simulink model "part2"  (R2022b)
settings: Solver=FixedStepAuto  StartTime=0.0  StopTime=500  FixedStep=0.1  RelTol=1e-3
values from neighbouring files (symbols this model uses):
  beta_c = 270    [init.m]
  D = [2.6486e5 0 0; 0 8.8164e5 0; 0 0 3.3774e8]    [KalmanKladd.m]    (also in init.m)
  init_setPoint = [0 0 0]    [init.m]
  K1 = [diag([k_1,k_2,k_3]) ... (first row only)    [init.m]
  K2 = diag([k_7,k_8,k_9])    [init.m]
  K3 = 0.05*K4    [init.m]
  K4 = diag([diag(M)])    [init.m]
  Kd = [7e6 7e6 1e9]    [init.m]
  Ki = [1e3 3e5 1e6]    [init.m]
  Kp = [4e6 4e6 2e8]    [init.m]
  M = [6.8177e6 0 0; 0 7.8784e6 -2.5955e6; 0 -2.5955e6 3.57e9]    [KalmanKladd.m]    (also in init.m)
  omg2 = omg.*omg    [init.m]
  satMax = [3 3 0.05]    [init.m]
  setPoint0 = [0 0 0]    [init.m]
  setPoint1 = [50 0 0]    [init.m]
  setPoint2 = [50 -50 0]    [init.m]
  setPoint3 = [50 -50 -pi/4]    [init.m]
  setPoint4 = [0 -50 -pi/4]    [init.m]
  setPoint5 = [0 0 0]    [init.m]
  setPoint_change_time = 100    [init.m]
  setPoint_sim12 = [0 0 0]    [init.m]
  setPoint_sim3 = [10 10 3*pi/2]    [init.m]
  switch_condition = 0    [init.m]
  thrusters =     [thrusters_sup.mat]
  V_c = 0.2    [init.m]
  vessel =     [thrusters_sup.mat]
  Z2omg = 2*omg.*zeta    [init.m]
undefined symbols (not defined in the file or in its folder): A_w, C_w, Hoerner, T
libraries: marine_gnc x7, marine_hydro x2, simulink x1
settings Model: Creator=jonbjor  LastModifiedBy=Petter
settings SolverCC: AlgebraicLoopSolver=TrustRegion
settings DataIOCC: ReturnWorkspaceOutputs=off
settings DebuggingCC: UnconnectedInputMsg=warning  UnconnectedOutputMsg=warning  UnconnectedLineMsg=warning  SFMachineParentedDataDiag=warning  ArithmeticOperatorsInVariantConditions=warning
settings ModelReferenceCC: EnableRefExpFcnMdlSchedulingChecks=on
settings SFSimCC: SimUseLocalCustomCode=off  CustomCodeUndefinedFunction=UseInterfaceOnly
settings RTWCC: RTWUseLocalCustomCode=off

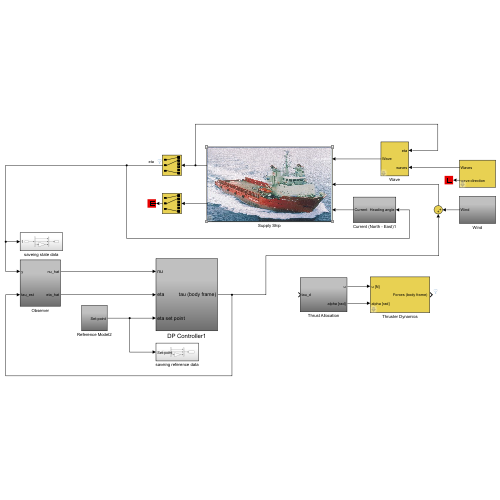
[thumbnail: Simulink's stored preview of the top-level diagram]
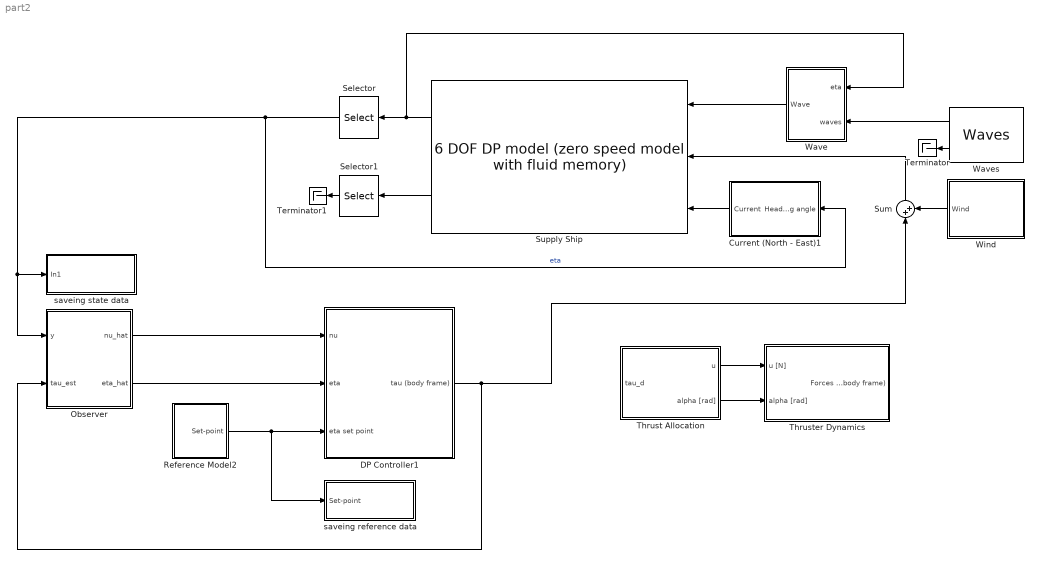
== system part2 ==
  Current (North - East)1 : Subsystem
  DP Controller1 : Subsystem
  Observer : Subsystem
  Reference Model2 : Subsystem
  Selector : Selector  InputPortWidth=6  IndexOptions=Index vector (dialog)  Indices=[1 2 6]  OutputSizes=1
  Selector1 : Selector  InputPortWidth=6  IndexOptions=Index vector (dialog)  Indices=[1 2 6]  OutputSizes=1
  Sum : Sum  Inputs=|++
  Supply Ship : marine_hydro/Hydro Library/6 DOF DP model  (zero speed model with fluid memory)  ABC=vesselABC  rho=1025  Axc=0.9*vessel.main.T*vessel.main.B  Ayc=0.9*vessel.main.T*vessel.main.Lpp  CX=1  CY_2D=Hoerner(vessel.main.B,vessel.main.T)  Bv=vessel.Bv  mask(6 DOF zero speed model){}
      link override "Integrator1 ": InitialCondition=nu0
      link override Integrator2: InitialCondition=eta0
      settings: SourceProductName=MSS Hydro
      mask Display:
      | image('supply.jpg');
      | color('white'); port_label('output', 1, 'eta')
      | color('white'); port_label('output', 2, 'nu')
      | color('white'); port_label('input', 1, 'tau_wave')
      | color('white'); port_label('input', 2, 'tau')
      | color('white'); port_label('input', 3, 'nu_c')
  Terminator : Terminator
  Terminator1 : Terminator
  Thrust Allocation : Subsystem
  Thruster Dynamics : Subsystem  mask{thrusterfault=off}
      mask prompts: thrusterfault "Fault on thruster #2 and #5?"
  Wave : Subsystem  mask{waveforces=on}
      mask prompts: waveforces "Waveforces enabled"
  Waves : marine_gnc/Environment/Waves/Waves  spectrum_type=ITTC  disp_flag=on  plot_spectrum=off  plot_realization=off  hs=5  omega_peak=pi/10  psi_mean=0  gamma=-1  spread=2  depth=inf  nfreq=20  ndir=10  energylim=0.005  freq_cutoff=3  dir_cutoff=0  rand_seed=123  rand_freq=on  rand_dir=on  Zeta_a=0  Omega=0  Phase=0  Wavenum=0  Psi=0
      settings: SourceProductName=MSS GNC
  Wind : Subsystem
  saveing reference data : Subsystem
  saveing state data : Subsystem
  wires:
  Supply Ship/2 -> Selector1/1
  Supply Ship/1 -> Wave/1(eta), Selector/1
  Wave/1(Wave) -> Supply Ship/1
  Waves/1 -> Wave/2(waves)
  Waves/2 -> Terminator/1
  Selector1/1 -> Terminator1/1
  Thrust Allocation/1(u) -> Thruster Dynamics/1(u [N])
  Wind/1(Wind) -> Sum/2
  DP Controller1/1(tau (body frame)) -> Observer/2(tau_est), Sum/1
  Sum/1 -> Supply Ship/2
  Thrust Allocation/2(alpha [rad]) -> Thruster Dynamics/2(alpha [rad])
  Selector/1 -> Current (North - East)1/1(Heading angle), saveing state data/1(In1), Observer/1(y)  "eta"
  Observer/2(eta_hat) -> DP Controller1/2(eta)
  Observer/1(nu_hat) -> DP Controller1/1(nu)
  Reference Model2/1(Set-point) -> saveing reference data/1(Set-point), DP Controller1/3(eta set point)
  Current (North - East)1/1(Current) -> Supply Ship/3

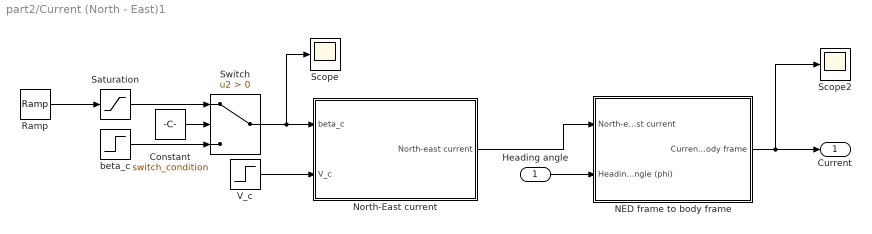
== system part2/Current (North - East)1 ==
  Heading angle : Inport
  Constant : Constant  Value=switch_condition
  NED frame to body frame : Subsystem
  North-East current : Subsystem
  Ramp : simulink/Sources/Ramp  slope=0.5  start=0  InitialOutput=0
  Saturation : Saturate  UpperLimit=90  LowerLimit=0
  Scope : Scope
  Scope2 : Scope
  Switch : Switch  Criteria=u2 > Threshold  SaturateOnIntegerOverflow=off  InputSameDT=off
  V_c : Step  Time=0  After=V_c  SampleTime=0
  beta_c : Step  Time=0  After=beta_c  SampleTime=0
  Current : Outport  VectorParamsAs1DForOutWhenUnconnected=off
  wires:
  V_c/1 -> North-East current/2(V_c)
  North-East current/1(North-east current) -> NED frame to body frame/1(North-east current)
  Heading angle/1 -> NED frame to body frame/2(Heading angle (phi))
  NED frame to body frame/1(Current body frame) -> Current/1, Scope2/1
  Ramp/1 -> Saturation/1
  Saturation/1 -> Switch/1
  Constant/1 -> Switch/2
  Switch/1 -> Scope/1, North-East current/1(beta_c)
  beta_c/1 -> Switch/3

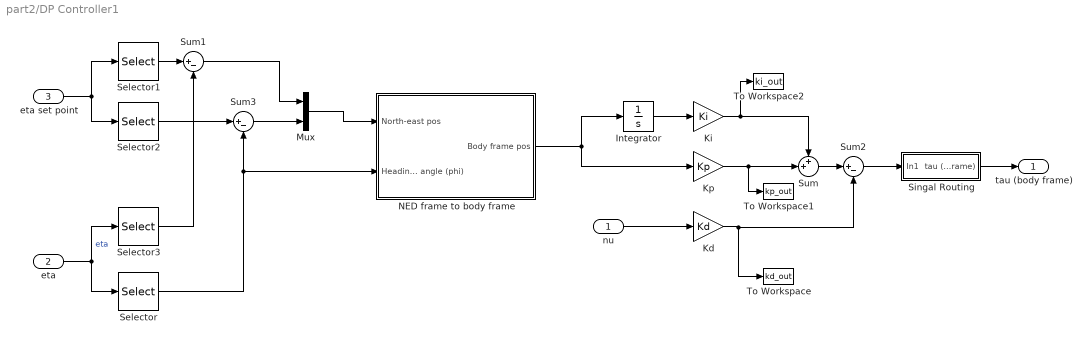
== system part2/DP Controller1 ==
  nu : Inport
  eta : Inport  Port=2
  eta set point : Inport  Port=3
  Integrator : Integrator
  Kd : Gain  Gain=Kd
  Ki : Gain  Gain=Ki
  Kp : Gain  Gain=Kp
  Mux : Mux  Inputs=2
  NED frame to body frame : Subsystem
  Selector : Selector  InputPortWidth=3  IndexOptions=Index vector (dialog)  Indices=[3]  OutputSizes=1
  Selector1 : Selector  InputPortWidth=3  IndexOptions=Index vector (dialog)  Indices=[1 2]  OutputSizes=1
  Selector2 : Selector  InputPortWidth=3  IndexOptions=Index vector (dialog)  Indices=[3]  OutputSizes=1
  Selector3 : Selector  InputPortWidth=3  IndexOptions=Index vector (dialog)  Indices=[1 2]  OutputSizes=1
  Singal Routing : Subsystem
  Sum : Sum  Inputs=++|
  Sum1 : Sum  Inputs=|+-
  Sum2 : Sum  Inputs=|+-
  Sum3 : Sum  Inputs=|+-
  To Workspace : ToWorkspace  VariableName=kd_out  SaveFormat=Timeseries  SampleTime=-1
  To Workspace1 : ToWorkspace  VariableName=kp_out  SaveFormat=Timeseries  SampleTime=-1
  To Workspace2 : ToWorkspace  VariableName=ki_out  SaveFormat=Timeseries  SampleTime=-1
  tau (body frame) : Outport  VectorParamsAs1DForOutWhenUnconnected=off
  wires:
  Kp/1 -> To Workspace1/1, Sum/2
  Ki/1 -> Sum/1, To Workspace2/1
  Kd/1 -> Sum2/2, To Workspace/1
  Integrator/1 -> Ki/1
  Sum/1 -> Sum2/1
  nu/1 -> Kd/1
  Sum2/1 -> Singal Routing/1(In1)
  Singal Routing/1(tau (body frame)) -> tau (body frame)/1
  NED frame to body frame/1(Body frame pos) -> Integrator/1, Kp/1
  eta set point/1 -> Selector2/1, Selector1/1
  eta/1 -> Selector/1, Selector3/1  "eta"
  Selector1/1 -> Sum1/1
  Selector3/1 -> Sum1/2
  Selector2/1 -> Sum3/1
  Selector/1 -> Sum3/2, NED frame to body frame/2(Heading angle (phi))
  Sum3/1 -> Mux/2
  Sum1/1 -> Mux/1
  Mux/1 -> NED frame to body frame/1(North-east pos)

== system part2/Observer ==
  y : Inport
  tau_est : Inport  Port=2
  Passive DP wave filter : marine_gnc/Navigation/Observers/Passive DP wave filter  lambda=0.1*diag([1 1 1])  w_o=diag([0.8 0.8 0.8])  K4=0.1*diag([1 1 0.1])  K3=0.1*diag([1 1 0.1])  w_c=1.3*diag([0.8 0.8 0.8])  T_b=diag([100 100 100])  M=diag([1 1 1])  D=diag([1 1 1])
      settings: SourceProductName=MSS GNC
  "Passive nonlinear observer " : Subsystem
  nu_hat : Outport  VectorParamsAs1DForOutWhenUnconnected=off
  eta_hat : Outport  Port=2  VectorParamsAs1DForOutWhenUnconnected=off
  wires:
  y/1 -> "Passive nonlinear observer "/1(y)
  tau_est/1 -> "Passive nonlinear observer "/2(tau_est)
  "Passive nonlinear observer "/1(nu_hat) -> nu_hat/1
  "Passive nonlinear observer "/2(eta_hat) -> eta_hat/1

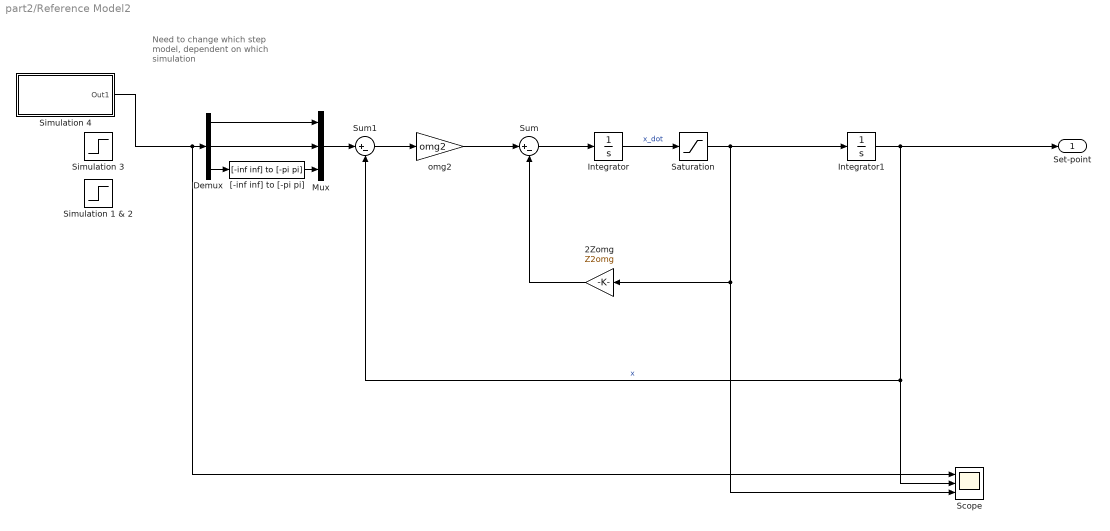
== system part2/Reference Model2 ==
  note: Need to change which step model, dependent on which simulation
  2Zomg : Gain  Gain=Z2omg
  Demux : Demux  Outputs=3
  Integrator : Integrator
  Integrator1 : Integrator
  Mux : Mux  Inputs=3
  Saturation : Saturate  UpperLimit=satMax  LowerLimit=-satMax
  Scope : Scope  NumInputPorts=3
  Simulation 1 & 2 : Step  Time=0  After=setPoint_sim12  SampleTime=0
  Simulation 3 : Step  Time=setPoint_change_time  Before=init_setPoint  After=setPoint_sim3  SampleTime=0
  Simulation 4 : Subsystem
  Sum : Sum  Inputs=|+-
  Sum1 : Sum  Inputs=|+-
  "[-inf inf] to [-pi pi]" : marine_gnc/Utilities/Math Operations/[-inf inf] to [-pi pi]
      settings: SourceProductName=MSS GNC
  omg2 : Gain  Gain=omg2
  Set-point : Outport  VectorParamsAs1DForOutWhenUnconnected=off
  wires:
  Integrator1/1 -> Set-point/1, Sum1/2, Scope/2  "x"
  Saturation/1 -> 2Zomg/1, Scope/3, Integrator1/1
  omg2/1 -> Sum/1
  Integrator/1 -> Saturation/1  "x_dot"
  Sum/1 -> Integrator/1
  Sum1/1 -> omg2/1
  2Zomg/1 -> Sum/2
  Simulation 4/1(Out1) -> Scope/1, Demux/1
  Mux/1 -> Sum1/1
  Demux/1 -> Mux/1
  Demux/2 -> Mux/2
  Demux/3 -> "[-inf inf] to [-pi pi]"/1
  "[-inf inf] to [-pi pi]"/1 -> Mux/3

== system part2/Thrust Allocation ==
  tau_d : Inport
  u : Outport  VectorParamsAs1DForOutWhenUnconnected=off
  alpha [rad] : Outport  Port=2  VectorParamsAs1DForOutWhenUnconnected=off

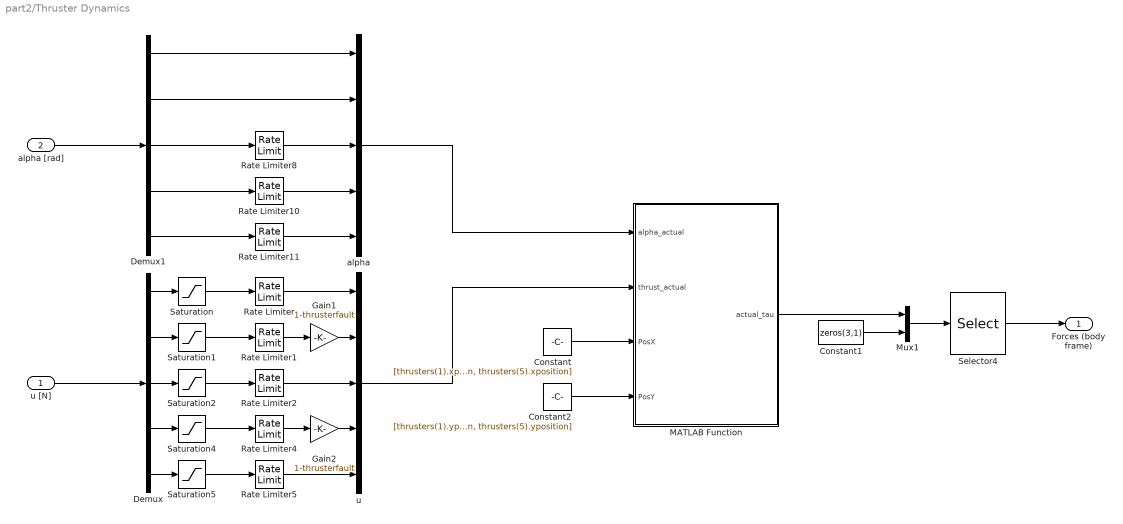
== system part2/Thruster Dynamics ==
  u [N] : Inport
  alpha [rad] : Inport  Port=2
  Constant : Constant  Value=[thrusters(1).xposition, thrusters(2).xposition, thrusters(3).xposition, thrusters(4).xposition, thrusters(5).xposition]
  Constant1 : Constant  Value=zeros(3,1)
  Constant2 : Constant  Value=[thrusters(1).yposition, thrusters(2).yposition, thrusters(3).yposition, thrusters(4).yposition, thrusters(5).yposition]
  Demux : Demux  Outputs=5
  Demux1 : Demux  Outputs=5
  Gain1 : Gain  Gain=1-thrusterfault
  Gain2 : Gain  Gain=1-thrusterfault
  MATLAB Function : MATLAB Function  TreatAsAtomicUnit=on
  Mux1 : Mux  Inputs=2
  Rate Limiter : RateLimiter  RisingSlewLimit=thrusters(1).rate  FallingSlewLimit=-thrusters(1).rate  SampleTimeMode=inherited
  Rate Limiter1 : RateLimiter  RisingSlewLimit=thrusters(2).rate  FallingSlewLimit=-thrusters(2).rate  SampleTimeMode=inherited
  Rate Limiter10 : RateLimiter  RisingSlewLimit=thrusters(4).rotationspeed  FallingSlewLimit=-thrusters(4).rotationspeed  SampleTimeMode=inherited
  Rate Limiter11 : RateLimiter  RisingSlewLimit=thrusters(5).rotationspeed  FallingSlewLimit=-thrusters(5).rotationspeed  SampleTimeMode=inherited
  Rate Limiter2 : RateLimiter  RisingSlewLimit=thrusters(3).rate  FallingSlewLimit=-thrusters(3).rate  SampleTimeMode=inherited
  Rate Limiter4 : RateLimiter  RisingSlewLimit=thrusters(4).rate  FallingSlewLimit=-thrusters(4).rate  SampleTimeMode=inherited
  Rate Limiter5 : RateLimiter  RisingSlewLimit=thrusters(5).rate  FallingSlewLimit=-thrusters(5).rate  SampleTimeMode=inherited
  Rate Limiter8 : RateLimiter  RisingSlewLimit=thrusters(3).rotationspeed  FallingSlewLimit=-thrusters(3).rotationspeed  SampleTimeMode=inherited
  Saturation : Saturate  UpperLimit=thrusters(1).thrust  LowerLimit=-thrusters(1).thrust
  Saturation1 : Saturate  UpperLimit=thrusters(2).thrust  LowerLimit=-thrusters(2).thrust
  Saturation2 : Saturate  UpperLimit=thrusters(3).thrust  LowerLimit=-thrusters(3).thrust
  Saturation4 : Saturate  UpperLimit=thrusters(4).thrust  LowerLimit=-thrusters(4).thrust
  Saturation5 : Saturate  UpperLimit=thrusters(5).thrust  LowerLimit=-thrusters(5).thrust
  Selector4 : Selector  InputPortWidth=6  IndexOptions=Index vector (dialog)  Indices=[1 2 4 5 6 3]  OutputSizes=1
  alpha : Mux  Inputs=5
  u : Mux  Inputs=5
  "Forces (body frame) " : Outport  VectorParamsAs1DForOutWhenUnconnected=off
  wires:
  Rate Limiter2/1 -> u/3
  Saturation/1 -> Rate Limiter/1
  Mux1/1 -> Selector4/1
  Constant1/1 -> Mux1/2
  Saturation4/1 -> Rate Limiter4/1
  Demux/2 -> Saturation1/1
  Saturation1/1 -> Rate Limiter1/1
  Demux/1 -> Saturation/1
  Demux/3 -> Saturation2/1
  Saturation2/1 -> Rate Limiter2/1
  Selector4/1 -> "Forces (body frame) "/1
  Gain1/1 -> u/2
  Rate Limiter1/1 -> Gain1/1
  Rate Limiter/1 -> u/1
  Rate Limiter4/1 -> Gain2/1
  Saturation5/1 -> Rate Limiter5/1
  Rate Limiter8/1 -> alpha/3
  u [N]/1 -> Demux/1
  alpha [rad]/1 -> Demux1/1
  Constant/1 -> MATLAB Function/3(PosX)
  Constant2/1 -> MATLAB Function/4(PosY)
  u/1 -> MATLAB Function/2(thrust_actual)
  alpha/1 -> MATLAB Function/1(alpha_actual)
  MATLAB Function/1(actual_tau) -> Mux1/1
  Demux1/3 -> Rate Limiter8/1
  Rate Limiter10/1 -> alpha/4
  Demux1/4 -> Rate Limiter10/1
  Demux1/5 -> Rate Limiter11/1
  Rate Limiter11/1 -> alpha/5
  Demux1/2 -> alpha/2
  Demux1/1 -> alpha/1
  Gain2/1 -> u/4
  Demux/4 -> Saturation4/1
  Demux/5 -> Saturation5/1
  Rate Limiter5/1 -> u/5

== system part2/Wave ==
  eta : Inport
  waves : Inport  Port=2
  Gain : Gain  Gain=waveforces
  Sum : Sum
  Wave loads (U=0) : marine_hydro/Hydro Library/Wave loads (U=0)  SystemSampleTime=-1  VariantActivationTime=update diagram  Latency=0  AutoFrameSizeCalculation=off
      settings: SourceProductName=MSS Hydro
  Wave : Outport  VectorParamsAs1DForOutWhenUnconnected=off
  wires:
  eta/1 -> Wave loads (U=0)/1
  waves/1 -> Wave loads (U=0)/2
  Sum/1 -> Gain/1
  Wave loads (U=0)/1 -> Sum/1
  Wave loads (U=0)/2 -> Sum/2
  Gain/1 -> Wave/1

== system part2/Wind ==
  Wind : Outport  VectorParamsAs1DForOutWhenUnconnected=off

== system part2/saveing reference data ==
  Set-point : Inport
  Demux : Demux  Outputs=3
  Gain : Gain  Gain=180/pi
  Mux : Mux  Inputs=3
  To Workspace2 : ToWorkspace  VariableName=set_point  SaveFormat=Timeseries  SampleTime=-1
  wires:
  Set-point/1 -> Demux/1
  Demux/1 -> Mux/1
  Demux/2 -> Mux/2
  Gain/1 -> Mux/3
  Demux/3 -> Gain/1
  Mux/1 -> To Workspace2/1

== system part2/saveing state data ==
  In1 : Inport
  Demux : Demux  Outputs=3
  Gain : Gain  Gain=180/pi
  Mux : Mux  Inputs=3
  To Workspace1 : ToWorkspace  VariableName=pos  SaveFormat=Timeseries  SampleTime=-1
  wires:
  In1/1 -> Demux/1
  Demux/1 -> Mux/1
  Demux/2 -> Mux/2
  Gain/1 -> Mux/3
  Demux/3 -> Gain/1
  Mux/1 -> To Workspace1/1

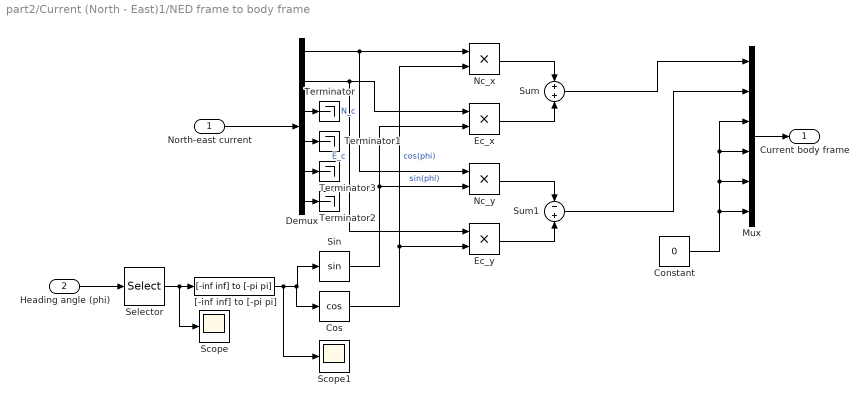
== system part2/Current (North - East)1/NED frame to body frame ==
  North-east current : Inport
  Heading angle (phi) : Inport  Port=2
  Constant : Constant  Value=0
  Cos : Trigonometry  Operator=cos
  Demux : Demux  Outputs=6
  Ec_x : Product
  Ec_y : Product
  Mux : Mux  Inputs=6
  Nc_x : Product
  Nc_y : Product
  Scope : Scope
  Scope1 : Scope
  Selector : Selector  InputPortWidth=3  IndexOptions=Index vector (dialog)  Indices=[3]  OutputSizes=1
  Sin : Trigonometry
  Sum : Sum
  Sum1 : Sum  Inputs=-+
  Terminator{,1..3} (4 alike) : Terminator
  "[-inf inf] to [-pi pi]" : marine_gnc/Utilities/Math Operations/[-inf inf] to [-pi pi]
      settings: SourceProductName=MSS GNC
  Current body frame : Outport
  wires:
  North-east current/1 -> Demux/1
  Demux/1 -> Nc_y/1, Nc_x/1  "N_c"
  Mux/1 -> Current body frame/1
  Cos/1 -> Ec_y/2, Nc_x/2  "cos(phi)"
  Demux/3 -> Terminator/1
  Demux/4 -> Terminator1/1
  Demux/6 -> Terminator2/1
  Demux/5 -> Terminator3/1
  Demux/2 -> Ec_y/1, Ec_x/1  "E_c"
  Sin/1 -> Nc_y/2, Ec_x/2  "sin(phi)"
  Ec_x/1 -> Sum/2
  Nc_x/1 -> Sum/1
  Sum/1 -> Mux/1
  Nc_y/1 -> Sum1/1
  Ec_y/1 -> Sum1/2
  Sum1/1 -> Mux/2
  Constant/1 -> Mux/6, Mux/5, Mux/4, Mux/3
  Heading angle (phi)/1 -> Selector/1
  Selector/1 -> Scope/1, "[-inf inf] to [-pi pi]"/1
  "[-inf inf] to [-pi pi]"/1 -> Scope1/1, Cos/1, Sin/1

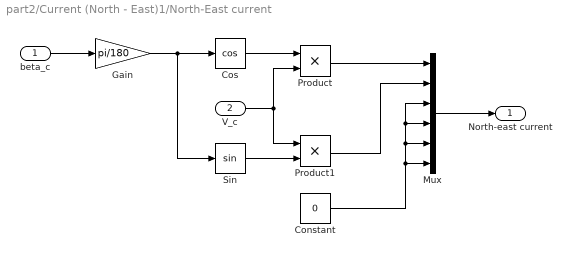
== system part2/Current (North - East)1/North-East current ==
  beta_c : Inport
  V_c : Inport  Port=2
  Constant : Constant  Value=0
  Cos : Trigonometry  Operator=cos
  Gain : Gain  Gain=pi/180
  Mux : Mux  Inputs=6
  Product : Product
  Product1 : Product
  Sin : Trigonometry
  North-east current : Outport
  wires:
  beta_c/1 -> Gain/1
  Gain/1 -> Sin/1, Cos/1
  Cos/1 -> Product/1
  V_c/1 -> Product1/1, Product/2
  Sin/1 -> Product1/2
  Product/1 -> Mux/1
  Product1/1 -> Mux/2
  Mux/1 -> North-east current/1
  Constant/1 -> Mux/6, Mux/5, Mux/4, Mux/3

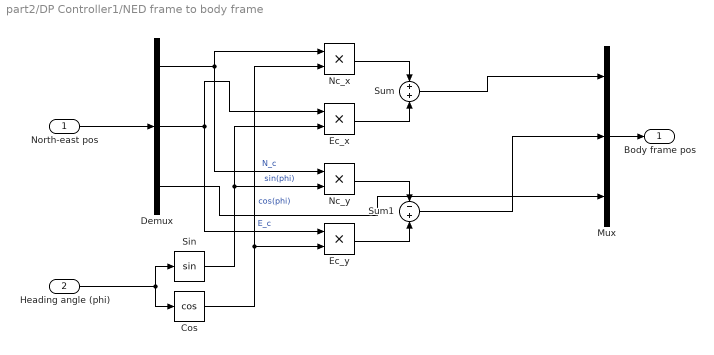
== system part2/DP Controller1/NED frame to body frame ==
  North-east pos : Inport
  Heading angle (phi) : Inport  Port=2
  Cos : Trigonometry  Operator=cos
  Demux : Demux  Outputs=3
  Ec_x : Product
  Ec_y : Product
  Mux : Mux  Inputs=3
  Nc_x : Product
  Nc_y : Product
  Sin : Trigonometry
  Sum : Sum
  Sum1 : Sum  Inputs=-+
  Body frame pos : Outport
  wires:
  North-east pos/1 -> Demux/1
  Demux/1 -> Nc_x/1, Nc_y/1  "N_c"
  Mux/1 -> Body frame pos/1
  Cos/1 -> Ec_y/2, Nc_x/2  "cos(phi)"
  Demux/2 -> Ec_y/1, Ec_x/1  "E_c"
  Sin/1 -> Nc_y/2, Ec_x/2  "sin(phi)"
  Ec_x/1 -> Sum/2
  Nc_x/1 -> Sum/1
  Sum/1 -> Mux/1
  Nc_y/1 -> Sum1/1
  Ec_y/1 -> Sum1/2
  Sum1/1 -> Mux/2
  Heading angle (phi)/1 -> Sin/1, Cos/1
  Demux/3 -> Mux/3

== system part2/DP Controller1/Singal Routing ==
  In1 : Inport
  Constant : Constant  Value=0
  Demux : Demux  Outputs=3
  Mux : Mux  Inputs=6
  tau (body frame) : Outport
  wires:
  Demux/1 -> Mux/1
  Constant/1 -> Mux/3, Mux/5, Mux/4
  In1/1 -> Demux/1
  Demux/2 -> Mux/2
  Mux/1 -> tau (body frame)/1
  Demux/3 -> Mux/6

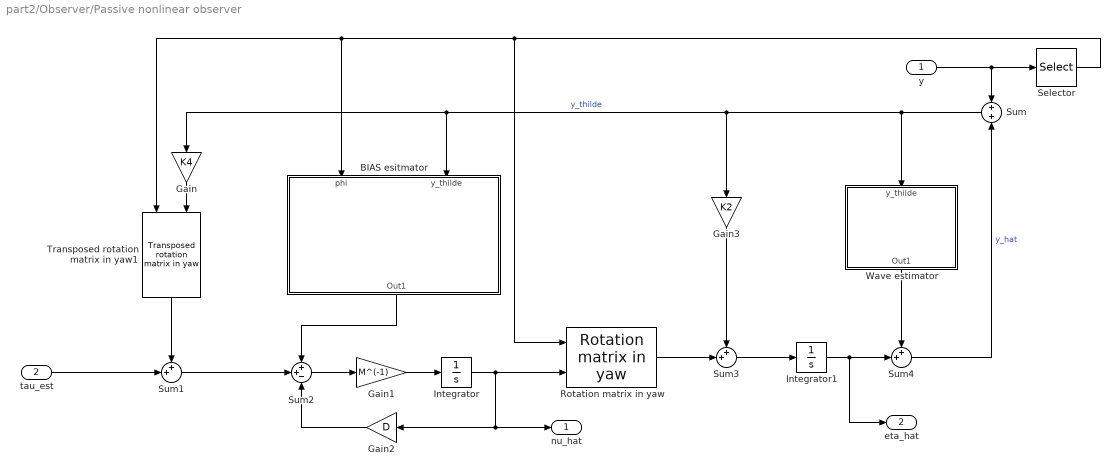
== system part2/Observer/Passive nonlinear observer  ==
  y : Inport
  tau_est : Inport  Port=2
  BIAS esitmator : Subsystem
  Gain : Gain  Gain=K4
  Gain1 : Gain  Gain=M^(-1)
  Gain2 : Gain  Gain=D
  Gain3 : Gain  Gain=K2
  Integrator : Integrator
  Integrator1 : Integrator
  "Rotation matrix in yaw " : marine_gnc/Models/ Kinematics/Rotation matrix in yaw 
      settings: SourceProductName=MSS GNC
  Selector : Selector  InputPortWidth=3  IndexOptions=Index vector (dialog)  Indices=[3]  OutputSizes=1
  Sum : Sum
  Sum1 : Sum  Inputs=++|
  Sum2 : Sum  Inputs=++-
  Sum3 : Sum  Inputs=++|
  Sum4 : Sum  Inputs=++|
  Transposed rotation matrix in yaw1 : marine_gnc/Models/ Kinematics/Transposed rotation  matrix in yaw
      settings: SourceProductName=MSS GNC
  Wave estimator : Subsystem
  nu_hat : Outport  VectorParamsAs1DForOutWhenUnconnected=off
  eta_hat : Outport  Port=2  VectorParamsAs1DForOutWhenUnconnected=off
  wires:
  Sum3/1 -> Integrator1/1
  Sum1/1 -> Sum2/2
  Gain1/1 -> Integrator/1
  tau_est/1 -> Sum1/2
  Gain3/1 -> Sum3/1
  Selector/1 -> Transposed rotation matrix in yaw1/1, BIAS esitmator/1(phi), "Rotation matrix in yaw "/1
  BIAS esitmator/1(Out1) -> Sum2/1
  Integrator/1 -> Gain2/1, nu_hat/1, "Rotation matrix in yaw "/2
  Transposed rotation matrix in yaw1/1 -> Sum1/1
  Integrator1/1 -> eta_hat/1, Sum4/2
  Sum2/1 -> Gain1/1
  y/1 -> Selector/1, Sum/1
  Wave estimator/1(Out1) -> Sum4/1
  Gain/1 -> Transposed rotation matrix in yaw1/2
  "Rotation matrix in yaw "/1 -> Sum3/2
  Sum4/1 -> Sum/2  "y_hat"
  Gain2/1 -> Sum2/3
  Sum/1 -> Wave estimator/1(y_thilde), Gain3/1, Gain/1, BIAS esitmator/2(y_thilde)  "y_thilde"

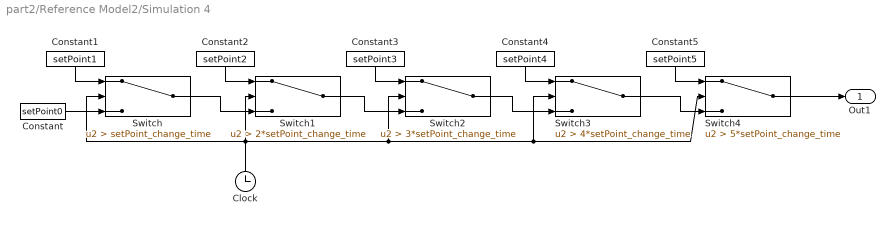
== system part2/Reference Model2/Simulation 4 ==
  Clock : Clock
  Constant : Constant  Value=setPoint0
  Constant1 : Constant  Value=setPoint1
  Constant2 : Constant  Value=setPoint2
  Constant3 : Constant  Value=setPoint3
  Constant4 : Constant  Value=setPoint4
  Constant5 : Constant  Value=setPoint5
  Switch : Switch  Criteria=u2 > Threshold  Threshold=setPoint_change_time  SaturateOnIntegerOverflow=off  InputSameDT=off
  Switch1 : Switch  Criteria=u2 > Threshold  Threshold=2*setPoint_change_time  SaturateOnIntegerOverflow=off  InputSameDT=off
  Switch2 : Switch  Criteria=u2 > Threshold  Threshold=3*setPoint_change_time  SaturateOnIntegerOverflow=off  InputSameDT=off
  Switch3 : Switch  Criteria=u2 > Threshold  Threshold=4*setPoint_change_time  SaturateOnIntegerOverflow=off  InputSameDT=off
  Switch4 : Switch  Criteria=u2 > Threshold  Threshold=5*setPoint_change_time  SaturateOnIntegerOverflow=off  InputSameDT=off
  Out1 : Outport
  wires:
  Constant/1 -> Switch/3
  Switch/1 -> Switch1/3
  Constant2/1 -> Switch1/1
  Switch1/1 -> Switch2/3
  Constant4/1 -> Switch3/1
  Switch2/1 -> Switch3/3
  Switch3/1 -> Switch4/3
  Clock/1 -> Switch3/2, Switch4/2, Switch2/2, Switch/2, Switch1/2
  Constant3/1 -> Switch2/1
  Constant5/1 -> Switch4/1
  Switch4/1 -> Out1/1
  Constant1/1 -> Switch/1

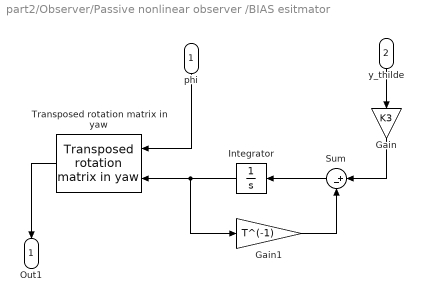
== system part2/Observer/Passive nonlinear observer /BIAS esitmator ==
  phi : Inport
  y_thilde : Inport  Port=2
  Gain : Gain  Gain=K3
  Gain1 : Gain  Gain=T^(-1)
  Integrator : Integrator
  Sum : Sum  Inputs=|+-
  Transposed rotation matrix in yaw : marine_gnc/Models/ Kinematics/Transposed rotation  matrix in yaw
      settings: SourceProductName=MSS GNC
  Out1 : Outport
  wires:
  y_thilde/1 -> Gain/1
  Gain/1 -> Sum/1
  Sum/1 -> Integrator/1
  Gain1/1 -> Sum/2
  Integrator/1 -> Transposed rotation matrix in yaw/2, Gain1/1
  phi/1 -> Transposed rotation matrix in yaw/1
  Transposed rotation matrix in yaw/1 -> Out1/1

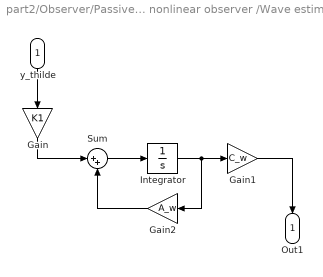
== system part2/Observer/Passive nonlinear observer /Wave estimator ==
  y_thilde : Inport
  Gain : Gain  Gain=K1
  Gain1 : Gain  Gain=C_w
  Gain2 : Gain  Gain=A_w
  Integrator : Integrator
  Sum : Sum  Inputs=|++
  Out1 : Outport
  wires:
  y_thilde/1 -> Gain/1
  Integrator/1 -> Gain2/1, Gain1/1
  Sum/1 -> Integrator/1
  Gain/1 -> Sum/1
  Gain2/1 -> Sum/2
  Gain1/1 -> Out1/1

== matlab function part2/Thruster Dynamics/MATLAB Function ==
  data: alpha_actual input; thrust_actual input; actual_tau output; PosX input; PosY input
function actual_tau   = fcn(alpha_actual,thrust_actual,PosX,PosY)

    Alpha_surge =[cos(alpha_actual(1)) cos(alpha_actual(2)) cos(alpha_actual(3)) cos(alpha_actual(4)) cos(alpha_actual(5))];  
    Alpha_sway = [sin(alpha_actual(1)) sin(alpha_actual(2)) sin(alpha_actual(3)) sin(alpha_actual(4)) sin(alpha_actual(5))];
    Alpha_yaw = [sin(alpha_actual(1))*PosX(1)-cos(alpha_actual(1))*PosY(1) sin(alpha_actual(2))*PosX(2)-cos(alpha_actual(2))*PosY(2) ...
                 sin(alpha_actual(3))*PosX(3)-cos(alpha_actual(3))*PosY(3) sin(alpha_actual(4))*PosX(4)-cos(alpha_actual(4))*PosY(4) ...
                 sin(alpha_actual(5))*PosX(5)-cos(alpha_actual(5))*PosY(5)];

    actual_tau = [Alpha_surge; Alpha_sway; Alpha_yaw]*thrust_actual;
end
